simulink model "door_le"  (R2014a)
settings: Solver=FixedStepDiscrete  StartTime=0.0  StopTime=1000.0  RelTol=1e-3
PostLoadFcn:
  | % check whether version is 9.1 (2016b) or newer
  | % and uncheck the multitasking checkbox
  | % as this checkbox is checked by default
  | if ~verLessThan('matlab', '9.1')
  |   set_param(bdroot, 'EnableMultiTasking','off');
  | end
undefined symbols (not defined in the file): DiscIntNeverNeededParam
libraries: canoelib x5, simulink x1
settings Model: ExtModeTrigMode=oneshot  ExtModeArmWhenConnect=off  Creator=vismrr  LastModifiedBy=vikafla
settings DataIOCC: LimitDataPoints=off  SignalLoggingSaveFormat=ModelDataLogs
settings OptimizationCC: BlockReduction=off  BooleanDataType=off  ExpressionDepthLimit=2147483647  InitFltsAndDblsToZero=on
settings DebuggingCC: SaveWithParameterizedLinksMsg=none  UnderspecifiedInitializationDetection=Classic  SignalResolutionControl=TryResolveAllWithWarning  SolverPrmCheckMsg=none  MultiTaskDSMMsg=warning  MultiTaskCondExecSysMsg=none  FcnCallInpInsideContextMsg=EnableAllAsWarning  StateNameClashWarn=warning  StrictBusMsg=None
settings HardwareCC: TargetLongLongMode=on  TargetIntDivRoundTo=Zero  TargetEndianess=LittleEndian  TargetHWDeviceType=MATLAB Host  ProdEqTarget=off
settings RTWCC: SystemTargetFile=cn.tlc  TemplateMakefile=cn_msdll.tmf  ProcessScript=cn_make_rtw_hook  IncludeERTFirstTime=on
settings STFCustomTargetCC: ConcurrentExecutionCompliant=off  MatFileLogging=on  CPPClassGenCompliant=on  SystemTargetFile=cn.tlc
settings GRTTargetCC: ParMdlRefBuildCompliant=off  CompOptLevelCompliant=off  ConcurrentExecutionCompliant=off  CombineOutputUpdateFcns=off  GRTInterface=on  ExtModeMexFile=noextcomm  RTWCAPISignals=on  RTWCAPIParams=on

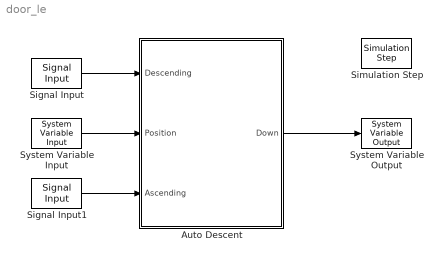
== system door_le ==
  Auto Descent : Subsystem
  Signal Input : canoelib/CANoe I//O/Signal Input  dbName=""  nodeName=""  msgName=""  sigName=WN_left_down  editSampleTime=0  rawValue=Physical value  dataType=Default  dataTypeDB=unknown  hasEncoding=off
      settings: AttributesFormatString=%<sigName>
  Signal Input1 : canoelib/CANoe I//O/Signal Input  dbName=""  nodeName=""  msgName=""  sigName=WN_left_up  editSampleTime=0  rawValue=Physical value  dataType=Default  dataTypeDB=unknown  hasEncoding=off
      settings: AttributesFormatString=%<sigName>
  Simulation Step : canoelib/CANoe I//O/Simulation Step  mode=Offline
      settings: AttributesFormatString=%<mode>
  System Variable Input : canoelib/CANoe I//O/System Variable Input  nsName=Door_Le  sysVarName=WN_Position  arrayIndex=-1  editSampleTime=0  rawValue=Default  dataType=Default  dataTypeDB=unknown  hasEncoding=off  dataTypeCANoe=Get from CANoe
      settings: AttributesFormatString=%<nsName>::%<sysVarName>
  System Variable Output : canoelib/CANoe I//O/System Variable Output  nsName=Door_Le  sysVarName=WN_Down  arrayIndex=-1  rawValue=Default  dataType=Default  dataTypeDB=unknown  hasEncoding=off  dataTypeCANoe=Get from CANoe
      settings: AttributesFormatString=%<nsName>::%<sysVarName>
  wires:
  System Variable Input/1 -> Auto Descent/2(Position)
  Signal Input/1 -> Auto Descent/1(Descending)
  Signal Input1/1 -> Auto Descent/3(Ascending)
  Auto Descent/1(Down) -> System Variable Output/1

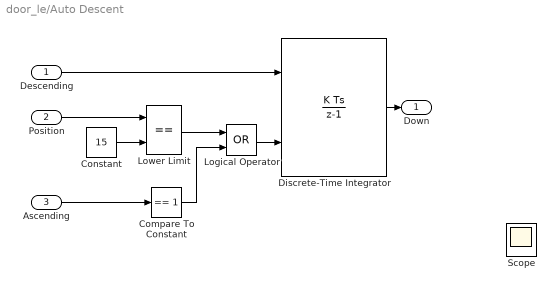
== system door_le/Auto Descent ==
  Descending : Inport
  Position : Inport  Port=2
  Ascending : Inport  Port=3
  Compare To Constant : simulink/Logic and Bit Operations/Compare To Constant  SystemSampleTime=-1  relop===  const=1  LogicOutDataTypeMode=uint8
  Constant : Constant  Value=15
  Discrete-Time Integrator : DiscreteIntegrator  gainval=2  ExternalReset=rising  SampleTime=0.01  LimitOutput=on  UpperSaturationLimit=1  LowerSaturationLimit=0  ICPrevOutput=DiscIntNeverNeededParam  ICPrevScaledInput=DiscIntNeverNeededParam
  Logical Operator : Logic  Operator=OR  AllPortsSameDT=off  OutDataTypeStr=boolean
  Lower Limit : RelationalOperator  Operator===  InputSameDT=on
  Scope : Scope  NumInputPorts=2
      settings: YMin=-1~14.25  YMax=1~15.75
  Down : Outport
  wires:
  Discrete-Time Integrator/1 -> Down/1
  Descending/1 -> Discrete-Time Integrator/1
  Constant/1 -> Lower Limit/2
  Position/1 -> Lower Limit/1
  Logical Operator/1 -> Discrete-Time Integrator/2
  Lower Limit/1 -> Logical Operator/1
  Ascending/1 -> Compare To Constant/1
  Compare To Constant/1 -> Logical Operator/2
